simulink model "testPID"  (R2024b)
settings: Solver=FixedStepAuto  StartTime=0.0  StopTime=10.0  RelTol=1e-3
undefined symbols (not defined in the file): kd, ki, kp, maxVoltage, minVoltage
settings Model: Creator=felipe  LastModifiedBy=felipe
settings OptimizationCC: PassReuseOutputArgsAs=Individual arguments  OptimizeBlockOrder=speed  DifferentSizesBufferReuse=on  EfficientTunableParamExpr=on
settings DebuggingCC: ParameterTunabilityLossMsg=error
settings HardwareCC: TargetBitPerLong=64  TargetBitPerPointer=64  TargetBitPerSizeT=64  TargetBitPerPtrDiffT=64  TargetLongLongMode=on  TargetIntDivRoundTo=Zero  TargetEndianess=LittleEndian  TargetWordSize=64  TargetHWDeviceType=MATLAB Host  ProdEqTarget=off
settings SFSimCC: MATLABDynamicMemAlloc=off
settings RTWCC: Description=Embedded Coder (host-based shared library target)  SystemTargetFile=ert_shrlib.tlc  TemplateMakefile=ert_default_tmf  RTWVerbose=off
settings RTWCC: CustomSourceCode=|
  | #define CONCAT(str1, str2, str3) CONCAT_(str1, str2, str3)
  | #define CONCAT_(str1, str2, str3) str1 ## str2 ## str3
  | #define GET_MMI_FUNC    CONCAT(MODEL     , _GetCAPImmi ,    )
  | #define RT_MODEL_STRUCT CONCAT(RT_MODEL_ , MODEL       , _T )
  | 
  | void* GET_MMI_FUNC(void* voidPtrToRealTimeStructure)
  | {
  |    rtwCAPI_ModelMappingInfo* mmiPtr = &(rtmGetDataMapInfo( ( RT_MODEL_STRUCT * )(voidPtrToRealTimeStructure) ).mmi);
  |    return (void*) mmiPtr;
  | }
settings CodeAppCC: GenerateComments=off  IgnoreCustomStorageClasses=off  OperatorAnnotations=on  SimulinkDataObjDesc=on  SFDataObjDesc=on  SimulinkBlockComments=off
settings STFCustomTargetCC: TargetLangStandard=C99 (ISO)  MultiwordLength=256  ParMdlRefBuildCompliant=on  CompOptLevelCompliant=on  IncludeMdlTerminateFcn=off  CombineOutputUpdateFcns=on  CombineSignalStateStructs=on  SuppressErrorStatus=on  ERTCustomFileBanners=on  SupportAbsoluteTime=off  CodeInterfacePackaging=Reusable function  SupportComplex=off  SupportContinuousTime=off  SupportNonInlinedSFcns=off  RemoveResetFunc=on  MATLABClassNameForMDSCustomization=Simulink.SoftwareTarget.ERTCustomization  ModelStepFunctionPrototypeControlCompliant=on  GenerateAllocFcn=on  UseToolchainInfoCompliant=on  SystemTargetFile=ert_shrlib.tlc
settings ERTTargetCC: TargetLangStandard=C99 (ISO)  ConcurrentExecutionCompliant=off  IncludeMdlTerminateFcn=off  CombineSignalStateStructs=on  SuppressErrorStatus=on  SupportAbsoluteTime=off  CodeInterfacePackaging=Reusable function  SupportComplex=off  CPPClassGenCompliant=off  GenerateAllocFcn=on  InlinedParameterPlacement=Hierarchical  RootIOFormat=Part of model data structure  RTWCAPIParams=on  RTWCAPIRootIO=on  ERTCustomFileTemplate=example_file_process.tlc

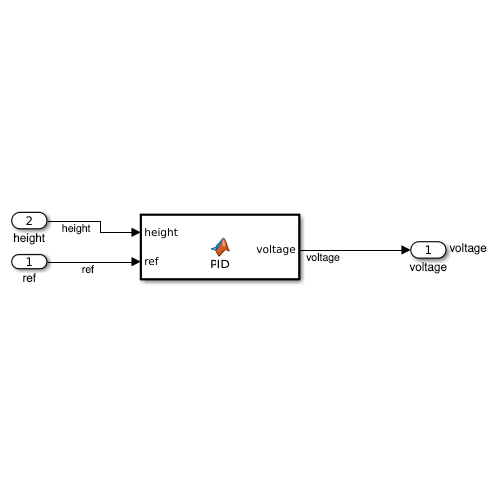
[thumbnail: Simulink's stored preview of the top-level diagram]
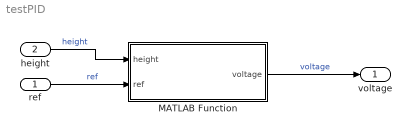
== system testPID ==
  ref : Inport
  height : Inport  Port=2
  MATLAB Function : MATLAB Function  TreatAsAtomicUnit=on
  voltage : Outport  SignalName=voltage
  wires:
  ref/1 -> MATLAB Function/2(ref)  "ref"
  height/1 -> MATLAB Function/1(height)  "height"
  MATLAB Function/1(voltage) -> voltage/1  "voltage"

== matlab function testPID/MATLAB Function ==
  data: height input; voltage output; ref input; kp parameter; ki parameter; kd parameter; maxVoltage parameter; minVoltage parameter; sampletime parameter
function voltage = PID(height, ref, kp, ki, kd, maxVoltage, minVoltage, sampletime)

persistent sum lastError enableIntegral lastIntegral kid kdd
if isempty(sum)
    sum = 0;
    lastError = 0;
    lastIntegral = 0;
    kid = ki * sampletime;
    kdd = kd / sampletime;
    enableIntegral = true;
end

error = ref - height;

proportional = kp * error;

if enableIntegral
    integral = (error * kid) + lastIntegral;
else
    integral = error * kid;
end

derivative = (error - lastError) * kdd;

voltage = proportional + integral + derivative;

lastError = error;
lastIntegral = integral;

% Anti-windup
if voltage > maxVoltage
    voltage = maxVoltage;
    enableIntegral = false;
elseif voltage < minVoltage
    voltage = minVoltage;
    enableIntegral = false;
else
    enableIntegral = true;
end

end
